simulink model "BimanualHD2LfD_2017a"  (R2017a)
settings: Solver=ode1  StartTime=0.0  StopTime=inf  FixedStep=0.002  RelTol=1e-3  EnableMultiTasking=on
undefined symbols (not defined in the file or in its folder): HIL, qc_get_step_size
libraries: quarc_library x10, simulink_extras x4, dsparch4 x3, simulink x2
(part 2 of 2)

== system BimanualHD2LfD_2017a/HD2 Dynamics/Endonesial I//O/HIL Interfacing/Subsystem1 ==
  Constant2 : Constant  Value=0.01
  Data Type Conversion : DataTypeConversion
  Data Type Conversion1 : DataTypeConversion
  De Bouncer : Subsystem
  De Bouncer1 : Subsystem
  Display : Display
  Display1 : Display
  HIL Read Digital : quarc_library/Data Acquisition/Generic/Immediate I//O/HIL Read Digital  object_name=HIL-1  channels=[0 1 7]  sample_time=qc_get_step_size  active=on  vector_output=off  data_type_mode=Inherit via back propagation  data_type=boolean
      settings: AttributesFormatString=(%<object_name>)
  Left : Outport
  Right : Outport  Port=2
  Touch Sensor : Outport  Port=3
  wires:
  HIL Read Digital/3 -> Touch Sensor/1
  HIL Read Digital/2 -> Display/1, Data Type Conversion1/1
  HIL Read Digital/1 -> Display1/1, Data Type Conversion/1
  Data Type Conversion/1 -> De Bouncer/1(Input)
  Data Type Conversion1/1 -> De Bouncer1/1(Input)
  Constant2/1 -> De Bouncer1/2(debounce_time), De Bouncer/2(debounce_time)
  De Bouncer/1(Output) -> Left/1
  De Bouncer1/1(Output) -> Right/1

== system BimanualHD2LfD_2017a/HD2 Dynamics/Endonesial I//O/HIL Interfacing/Subsystem1/De Bouncer ==
  Input : Inport
  debounce_time : Inport  Port=2
  Data Type Conversion : DataTypeConversion  OutDataTypeStr=int32
  Embedded MATLAB Function : MATLAB Function  TreatAsAtomicUnit=on
  Gain : Gain  Gain=1/qc_get_step_size
  Memory : Memory  InheritSampleTime=on  LinearizeMemory=on  LinearizeAsDelay=on
  Memory1 : Memory  InheritSampleTime=on  LinearizeMemory=on  LinearizeAsDelay=on
  Output : Outport
  wires:
  Embedded MATLAB Function/1(output) -> Memory/1, Output/1
  Embedded MATLAB Function/2(counter) -> Memory1/1
  Memory/1 -> Embedded MATLAB Function/3(prev_output)
  Memory1/1 -> Embedded MATLAB Function/4(prev_counter)
  Input/1 -> Embedded MATLAB Function/1(input)
  debounce_time/1 -> Gain/1
  Data Type Conversion/1 -> Embedded MATLAB Function/2(num_samples)
  Gain/1 -> Data Type Conversion/1

== system BimanualHD2LfD_2017a/HD2 Dynamics/Endonesial I//O/HIL Interfacing/Subsystem1/De Bouncer1 ==
  Input : Inport
  debounce_time : Inport  Port=2
  Data Type Conversion : DataTypeConversion  OutDataTypeStr=int32
  Embedded MATLAB Function : MATLAB Function  TreatAsAtomicUnit=on
  Gain : Gain  Gain=1/qc_get_step_size
  Memory : Memory  InheritSampleTime=on  LinearizeMemory=on  LinearizeAsDelay=on
  Memory1 : Memory  InheritSampleTime=on  LinearizeMemory=on  LinearizeAsDelay=on
  Output : Outport
  wires:
  Gain/1 -> Data Type Conversion/1
  Data Type Conversion/1 -> Embedded MATLAB Function/2(num_samples)
  debounce_time/1 -> Gain/1
  Input/1 -> Embedded MATLAB Function/1(input)
  Memory1/1 -> Embedded MATLAB Function/4(prev_counter)
  Memory/1 -> Embedded MATLAB Function/3(prev_output)
  Embedded MATLAB Function/2(counter) -> Memory1/1
  Embedded MATLAB Function/1(output) -> Output/1, Memory/1

== matlab function BimanualHD2LfD_2017a/GMR/MATLAB Function ==
  data: outputs output; data input; I_vars input; O_vars input; output_var output; model parameter
function [outputs, output_var] = GMR_3DOF (data, I_vars, O_vars, model) 
%#codegen
    [outputs, output_var, ~] = GMR(model, data, I_vars, O_vars);
end

== matlab function BimanualHD2LfD_2017a/Remove Orientation Jump/Remove Orientation Jump ==
  data: signal input; prevSignal input; out output; time input
function out = removeJump(signal, prevSignal, time)
persistent jumpType;
persistent jumpDistance;
persistent jumpCounter;


    if isempty(jumpType) || (time < 0.1)
        jumpType = 0;
        jumpDistance = 0;
        jumpCounter = 0;
    end

    if (signal - prevSignal) < -1
        jumpType = -1;
        jumpCounter = jumpCounter - 1;
        jumpDistance = signal-prevSignal;
        
    elseif (signal - prevSignal) > 1
        jumpType = 1;
        jumpCounter = jumpCounter + 1;
        jumpDistance = signal-prevSignal;
    end
    
    if jumpType == 1
        out = signal - jumpDistance*jumpCounter;
    elseif jumpType == -1
        out = signal + jumpDistance*jumpCounter;
    else
        out = signal;
    end
end

== matlab function BimanualHD2LfD_2017a/Remove Orientation Jump/Remove Orientation Jump1 ==
  data: signal input; prevSignal input; out output; time input
function out = removeJump(signal, prevSignal, time)
persistent jumpType;
persistent jumpDistance;
persistent jumpCounter;


    if isempty(jumpType) || (time < 0.1)
        jumpType = 0;
        jumpDistance = 0;
        jumpCounter = 0;
    end

    if (signal - prevSignal) < -1
        jumpType = -1;
        jumpCounter = jumpCounter - 1;
        jumpDistance = signal-prevSignal;
        
    elseif (signal - prevSignal) > 1
        jumpType = 1;
        jumpCounter = jumpCounter + 1;
        jumpDistance = signal-prevSignal;
    end
    
    if jumpType == 1
        out = signal - jumpDistance*jumpCounter;
    elseif jumpType == -1
        out = signal + jumpDistance*jumpCounter;
    else
        out = signal;
    end
end

== matlab function BimanualHD2LfD_2017a/Kalman Filter ==
  data: x_meas input; DataFilt output
function DataFilt = KalmanFilter(x_meas)
%#codegen
    % Process and sensor noise covariances
    Q =  0.00001;
    R =  1;

    % Initialize estimate and covariance predictions
    persistent x P;
    if (isempty(x) || isempty(P))
        x = -145;
        P = 1;
    end
    P = P + Q;
        
    % Update Kalman gain, and estimate and covariance based on gain
    K = P/(P+R);
    x = x+K*(x_meas-x);
    P = (1-K)*P;
    
    DataFilt = x;
end

== matlab function BimanualHD2LfD_2017a/Remove Orientation Jump/Remove Orientation Jump2 ==
  data: signal input; prevSignal input; out output; time input
function out = removeJump(signal, prevSignal, time)
persistent jumpType;
persistent jumpDistance;
persistent jumpCounter;


    if isempty(jumpType) || (time < 0.1)
        jumpType = 0;
        jumpDistance = 0;
        jumpCounter = 0;
    end

    if (signal - prevSignal) < -1
        jumpType = -1;
        jumpCounter = jumpCounter - 1;
        jumpDistance = signal-prevSignal;
        
    elseif (signal - prevSignal) > 1
        jumpType = 1;
        jumpCounter = jumpCounter + 1;
        jumpDistance = signal-prevSignal;
    end
    
    if jumpType == 1
        out = signal - jumpDistance*jumpCounter;
    elseif jumpType == -1
        out = signal + jumpDistance*jumpCounter;
    else
        out = signal;
    end
end

== matlab function BimanualHD2LfD_2017a/Velpocity Saturation/MATLAB Function ==
  data: v input; v_sat output
function v_sat = saturate(v)
%#codegen
spd = norm(v);
if spd > 99.999
    v_sat = v * 99.999 / spd;
else
    v_sat = v;
end

== matlab function BimanualHD2LfD_2017a/Velocity Decomposition/MATLAB Function ==
  data: velDes input; dirDes output; spdDes output
function [dirDes, spdDes] = fcn(velDes)
%#codegen
    spdDes = norm(velDes);
    if (spdDes > 0)
        dirDes = velDes / spdDes;
    else
        dirDes = [0; 0; 0];
    end
end

== matlab function BimanualHD2LfD_2017a/HD2 Dynamics/Embedded MATLAB Function ==
  data: EmergStop input; out output; u1 input
function out  = fcn(EmergStop,u1)
if EmergStop==0
out=u1;
else
 out=0*u1;
end;

== matlab function BimanualHD2LfD_2017a/HD2 Dynamics/Endonesial I//O/5BAR Linkage Kinematics (Upper)/OMNI Revised Kinematics ==
  data: M input; l1 input; l2 input; p output; l3 input; J output
function [p, J] = Five_Bar_Linkage_Kinematics (M, l1, l2, l3)
	R = l2*cos(M(2)) + l3*cos(M(3));
	x = cos(M(1))*R;
	y = sin(M(1))*R;
	z = l2*sin(M(2)) + l3*sin(M(3)) + l1;
	p = [x y z]';
	J1 = [-sin(M(1))*R      -cos(M(1))*l2*sin(M(2))     -cos(M(1))*l3*sin(M(3))];
	J2 = [cos(M(1))*R       -sin(M(1))*l2*sin(M(2))     -sin(M(1))*l3*sin(M(3))];
	J3 = [0                 l2*cos(M(2))                    l3*cos(M(3))];
	J = [J1;J2;J3];
end

== matlab function BimanualHD2LfD_2017a/HD2 Dynamics/Endonesial I//O/5BAR Linkage Kinematics (Lower)/OMNI Revised Kinematics ==
  data: M input; l1 input; l2 input; p output; l3 input; J output
function [p, J] = Five_Bar_Linkage_Kinematics (M, l1, l2, l3)
% CONSTANTS TO FIX ANGLE OFFSETS, MIGHT NEED TO BE CHANGED (JASON)
e1 = 0.6109; e2 = 1.3963; e3 = 1.6581;

R = l2*cos(M(2)) + l3*cos(M(3));
x = cos(M(1))*R;
y = sin(M(1))*R;
z = l2*sin(M(2)) + l3*sin(M(3)) + l1;
p = [x y z]';
J1 = [-sin(M(1))*R      -cos(M(1))*l2*sin(M(2))     -cos(M(1))*l3*sin(M(3))];
J2 = [cos(M(1))*R       -sin(M(1))*l2*sin(M(2))     -sin(M(1))*l3*sin(M(3))];
J3 = [0                 l2*cos(M(2))                    l3*cos(M(3))];
J = [J1;J2;J3];
end

== matlab function BimanualHD2LfD_2017a/HD2 Dynamics/Endonesial I//O/Calculate Orientation ==
  data: x_upper input; theta_x output; theta_y output; x_lower input; theta_z output; theta_z_p input; counterNew output; counterOld input; theta_z_out output
function [theta_x, theta_y, theta_z, counterNew, theta_z_out] = ...
	fcn(x_upper, x_lower, theta_z_p, counterOld)
	% This block supports the Embedded MATLAB subset.
	% See the help menu for details. 

	theta_x = atan2(x_upper(3) - x_lower(3), x_upper(2) - x_lower(2));
	theta_y = atan2(x_upper(1) - x_lower(1), x_upper(3) - x_lower(3));
	theta_z = atan2(x_upper(2) - x_lower(2), x_upper(1) - x_lower(1));

	counterNew = counterOld;

	if theta_z >= 0
		F1 = mod(theta_z, 2*pi);
		theta_z = F1;
	else
		F1 = mod(theta_z, -2*pi) + 2*pi;
		theta_z = F1;
	end

	d_theta_z = theta_z_p - theta_z;

	if abs(d_theta_z) > 5
		if d_theta_z > 0
		counterNew = counterOld + 1;
		end
		if d_theta_z < 0
		counterNew = counterOld - 1;
		end
	end
 
	theta_z_out = theta_z + 2*pi*counterNew;
end

== matlab function BimanualHD2LfD_2017a/HD2 Dynamics/Endonesial I//O/HD^2 New Kin new frame/New Numerical Kin ==
  data: q input; pos output; or output; ang output; poses output; Trans output; nn output; x output
 function [pos, or ,ang , poses, Trans, nn, x] = HDsquared_forwardkin(q)

    x = [0 0 0 0]';
    l = [220 40 125 22.25 250];
    ang = [0 0 0];
    
  
    nn = 0;
    while ( (norm(fnum(q,x,l)) > 0.0001) && nn <20)
      nn = nn+1;
        x = x - inv(Jnum(q,x,l))*fnum(q,x,l)';
    end
    
    
    
    pos = handlePos(q,x,l)';
    or = handleOr(q,x,l);
     
%     yaw = atan2 (or(2,1),or(1,1));   %AA
%     roll = atan2 ( or(3,2),or(3,3) );  %AA
%     pitch = atan2( -or(3,1), sqrt(  or(3,2)^2 + or(3,3)^2 ) ); %AA
%     
%     ang = [yaw;pitch;roll];  %AA
    
    pos_top = 250/2*(or(:,3))+pos;
    pos_bottom = -250/2*(or(:,3))+pos;
    poses = [pos_top;pos_bottom];
    
    Trans1 = cat(2,or,pos);
    Trans = cat(1,Trans1,[0 0 0 1]);
    
end


function val = fnum(q,x,l)

val = zeros(1,4); %AA
    q1 = q(1);
    q2 = q(2);
    q3 = q(3);
    q4 = q(4);
    q5 = q(5);
    q6 = q(6);
    
    l1 = l(1);
    l2 = l(2);
    l3 = l(3);
    l4 = l(4);
    l5 = l(5);
    
    alpha_u = x(1);
    theta_u = x(2);
    alpha_l = x(3);
    theta_l = x(4);
    
    t1 = pi / 0.4e1;
    t3 = cos(t1 + q1);
    t4 = sin(alpha_u);
    t5 = t3 * t4;
    t7 = cos(-t1 + q1);
    t8 = sin(theta_u);
    t9 = t7 * t8;
    t10 = cos(alpha_u);
    t11 = t9 * t10;
    t13 = cos(t1 + q4);
    t14 = sin(alpha_l);
    t15 = t13 * t14;
    t17 = cos(-t1 + q4);
    t18 = sin(theta_l);
    t19 = t17 * t18;
    t20 = cos(alpha_l);
    t21 = t19 * t20;
    t23 = cos(q3);
    t24 = t23 * t7;
    t25 = t24 * t4;
    t28 = sin(q3);
    t29 = cos(theta_u);
    t31 = t23 * t3 * t8 + t28 * t29;
    t32 = t31 * t10;
    t33 = cos(q6);
    t34 = t33 * t17;
    t35 = t34 * t14;
    t38 = sin(q6);
    t39 = cos(theta_l);
    t41 = t33 * t13 * t18 + t38 * t39;
    t42 = t41 * t20;
    t45 = cos(-t1 + q2);
    t56 = cos(-t1 + q5);
    t68 = cos(t1 + q2);
    t80 = cos(t1 + q5);
    val(1) = t5 + t11 - t15 - t21;
    val(2) = -t25 + t32 + t35 - t42;
    val(3) = t45 * l1 - t3 * l1 + (-t3 * t10 + t9 * t4) * l4 - (t5 + t11) * l5 / 0.2e1 - t56 * l1 + t13 * l1 - (-t13 * t20 + t19 * t14) * l4 - (t15 + t21) * l5 / 0.2e1;
    val(4) = t23 * t68 * l1 + t24 * l1 + (t24 * t10 + t31 * t4) * l4 - (-t25 + t32) * l5 / 0.2e1 - t33 * t80 * l1 - t34 * l1 - (t34 * t20 + t41 * t14) * l4 - (-t35 + t42) * l5 / 0.2e1;

end



function val2 = Jnum(q,x,l)
val2 = zeros(4,4); %AA
    q1 = q(1);
    q2 = q(2);
    q3 = q(3);
    q4 = q(4);
    q5 = q(5);
    q6 = q(6);
    
    l1 = l(1);
    l2 = l(2);
    l3 = l(3);
    l4 = l(4);
    l5 = l(5);
    
    
    alpha_u = x(1);
    theta_u = x(2);
    alpha_l = x(3);
    theta_l = x(4);
    
    t1 = pi / 0.4e1;
    t3 = cos(t1 + q1);
    t4 = cos(alpha_u);
    t7 = cos(-t1 + q1);
    t8 = sin(theta_u);
    t9 = t7 * t8;
    t10 = sin(alpha_u);
    t12 = t3 * t4 - t9 * t10;
    t13 = cos(theta_u);
    t14 = t7 * t13;
    t17 = cos(t1 + q4);
    t18 = cos(alpha_l);
    t21 = cos(-t1 + q4);
    t22 = sin(theta_l);
    t23 = t21 * t22;
    t24 = sin(alpha_l);
    t26 = -t17 * t18 + t23 * t24;
    t27 = cos(theta_l);
    t28 = t21 * t27;
    t30 = cos(q3);
    t31 = t30 * t7;
    t33 = t30 * t3;
    t35 = sin(q3);
    t37 = t33 * t8 + t35 * t13;
    t39 = -t31 * t4 - t37 * t10;
    t42 = t33 * t13 - t35 * t8;
    t43 = t42 * t4;
    t44 = cos(q6);
    t45 = t44 * t21;
    t47 = t44 * t17;
    t49 = sin(q6);
    t51 = t47 * t22 + t49 * t27;
    t53 = t45 * t18 + t51 * t24;
    t56 = t47 * t27 - t49 * t22;
    t57 = t56 * t18;
    val2(1,1) = t12;
    val2(1,2) = t14 * t4;
    val2(1,3) = t26;
    val2(1,4) = -t28 * t18;
    val2(2,1) = t39;
    val2(2,2) = t43;
    val2(2,3) = t53;
    val2(2,4) = -t57;
    val2(3,1) = (t3 * t10 + t9 * t4) * l4 - t12 * l5 / 0.2e1;
    val2(3,2) = t14 * t10 * l4 - t14 * t4 * l5 / 0.2e1;
    val2(3,3) = -(t17 * t24 + t23 * t18) * l4 + t26 * l5 / 0.2e1;
    val2(3,4) = -t28 * t24 * l4 - t28 * t18 * l5 / 0.2e1;
    val2(4,1) = (-t31 * t10 + t37 * t4) * l4 - t39 * l5 / 0.2e1;
    val2(4,2) = t42 * t10 * l4 - t43 * l5 / 0.2e1;
    val2(4,3) = -(-t45 * t24 + t51 * t18) * l4 + t53 * l5 / 0.2e1;
    val2(4,4) = -t56 * t24 * l4 - t57 * l5 / 0.2e1;

end

function val3 = handlePos(q,x,l)
 val3 = zeros(1,3);   %AA
    q1 = q(1);
    q2 = q(2);
    q3 = q(3);
    q4 = q(4);
    q5 = q(5);
    q6 = q(6);
    
    l1 = l(1);
    l2 = l(2);
    l3 = l(3);
    l4 = l(4);
    l5 = l(5);
    
    
    alpha_u = x(1);
    theta_u = x(2);
    alpha_l = x(3);
    theta_l = x(4);

    t1 = pi / 0.4e1;
    t3 = cos(-t1 + q2);
    t6 = cos(t1 + q1);
    t8 = cos(alpha_u);
    t11 = cos(-t1 + q1);
    t12 = sin(theta_u);
    t13 = t11 * t12;
    t14 = sin(alpha_u);
    t24 = cos(q3);
    t26 = cos(t1 + q2);
    t29 = t24 * t11;
    t34 = sin(q3);
    t35 = cos(theta_u);
    t37 = t24 * t6 * t12 + t34 * t35;
    t49 = t34 * t11;
    t55 = -t34 * t6 * t12 + t24 * t35;
    val3(1) = t3 * l1 - t6 * l1 + (-t6 * t8 + t13 * t14) * l4 - (t6 * t14 + t13 * t8) * l5 / 0.2e1;
    val3(2) = t24 * t26 * l1 + t29 * l1 + (t29 * t8 + t37 * t14) * l4 - (-t29 * t14 + t37 * t8) * l5 / 0.2e1;
    val3(3) = l3 - t34 * t26 * l1 - t49 * l1 + (-t49 * t8 + t55 * t14) * l4 - (t49 * t14 + t55 * t8) * l5 / 0.2e1;

end

function val4 = handleOr(q,x,l)
  val4 = zeros(3,3);  %AA 
    q1 = q(1);
    q2 = q(2);
    q3 = q(3);
    q4 = q(4);
    q5 = q(5);
    q6 = q(6);
    q7 = q(7);
    
    l1 = l(1);
    l2 = l(2);
    l3 = l(3);
    l4 = l(4);
    l5 = l(5);
    
    
    alpha_u = x(1);
    theta_u = x(2);
    alpha_l = x(3);
    theta_l = x(4);
    
    t1 = pi / 0.4e1;
    t3 = cos(-t1 + q1);
    t4 = cos(theta_u);
    t5 = t3 * t4;
    t6 = cos(q7);
    t9 = cos(t1 + q1);
    t10 = cos(alpha_u);
    t12 = sin(theta_u);
    t13 = t3 * t12;
    t14 = sin(alpha_u);
    t16 = -t9 * t10 + t13 * t14;
    t17 = sin(q7);
    t26 = cos(q3);
    t27 = t26 * t9;
    t29 = sin(q3);
    t31 = t27 * t4 - t29 * t12;
    t33 = t26 * t3;
    t37 = t27 * t12 + t29 * t4;
    t39 = t33 * t10 + t37 * t14;
    t48 = t29 * t9;
    t51 = -t48 * t4 - t26 * t12;
    t53 = t29 * t3;
    t57 = -t48 * t12 + t26 * t4;
    t59 = -t53 * t10 + t57 * t14;
    val4(1,1) = t5 * t6 + t16 * t17;
    val4(1,2) = -t5 * t17 + t16 * t6;
    val4(1,3) = t9 * t14 + t13 * t10;
    val4(2,1) = t31 * t6 + t39 * t17;
    val4(2,2) = -t31 * t17 + t39 * t6;
    val4(2,3) = -t33 * t14 + t37 * t10;
    val4(3,1) = t51 * t6 + t59 * t17;
    val4(3,2) = -t51 * t17 + t59 * t6;
    val4(3,3) = t53 * t14 + t57 * t10;

end

== matlab function BimanualHD2LfD_2017a/HD2 Dynamics/Endonesial I//O/HIL Interfacing/Subsystem1/De Bouncer/Embedded MATLAB Function ==
  data: input input; num_samples input int32; output output; prev_output input; prev_counter input int32; counter output int32
function [output, counter] = de_bouncer(input,  num_samples,prev_output, prev_counter)
if (prev_output ~= input)
    % Change detected
    counter = prev_counter - 1;
    if (counter == 0)
        output = input;
    else
        output = prev_output;
    end
else
    counter = num_samples;
    output = prev_output;
end

== matlab function BimanualHD2LfD_2017a/HD2 Dynamics/Endonesial I//O/HIL Interfacing/Subsystem1/De Bouncer1/Embedded MATLAB Function ==
  data: input input; num_samples input int32; output output; prev_output input; prev_counter input int32; counter output int32
function [output, counter] = de_bouncer(input,  num_samples,prev_output, prev_counter)
if (prev_output ~= input)
    % Change detected
    counter = prev_counter - 1;
    if (counter == 0)
        output = input;
    else
        output = prev_output;
    end
else
    counter = num_samples;
    output = prev_output;
end

== matlab function BimanualHD2LfD_2017a/HD2 Dynamics/Endonesial I//O/Torque to Force ==
  data: x_lower input; F_upper output; F_lower output; x_upper input; tau input; l11 input; l22 input
function [F_upper,F_lower] = fcn(x_lower,x_upper,tau,l11,l22)
% This block supports the Embedded MATLAB subset.
% See the help menu for details. 


%Initialization
F_upper=zeros(3,1);
F_lower=zeros(3,1);

if l11 == 0 
    sg1 = 1;
else
    sg1= sign(l11);
end

if l22 == 0 
    sg2 = 1;
else
    sg2= sign(l22);
end



if abs(l11)<0.005 
    l1 = 0.005 * sg1;
else
    l1= l11;
end

if abs(l22)<0.005 
    l2 = 0.005 * sg2;
else
    l2= l22;
end
%%%%%%%%%%%%%%%%%%%%%%%%%%%%

link = sqrt (  (x_upper(3)-x_lower(3))^2 + (x_upper(1)-x_lower(1))^2  + (x_upper(2)-x_lower(2))^2  );
unitvec = (x_upper - x_lower)/link;
F_upper = ( cross (tau,unitvec))/2/l1;
F_lower = - ( cross (tau,unitvec))/2/l2;


% link = sqrt (  (x_upper(3)-x_lower(3))^2 + (x_upper(1)-x_lower(1))^2  + (x_upper(2)-x_lower(2))^2  );
% unitvec = (x_upper - x_lower)/link;
% F_upper = 2/link * ( cross (tau,unitvec));
% F_lower = - F_upper;
% 

% link = sqrt (  (x_upper(3)-x_lower(3))^2 + (x_upper(1)-x_lower(1))^2  + (x_upper(2)-x_lower(2))^2  );
% unitvec = (x_lower - x_upper)/link;
% F_upper = (5/link * ( cross (tau,unitvec)));
% F_lower = F_upper/6;

== matlab function BimanualHD2LfD_2017a/HD2 Dynamics/Endonesial I//O/Calculate Mean Position ==
  data: x_mean output; x input; l1 input
function x_mean  = mean1(x,l1)
% This block supports the Embedded MATLAB subset.
% See the help menu for details. 
% link = .175;%25;
% l2=link - l1;
% 
% x_mean=zeros(3,1);
% x_mean(1)=(l2*x(1)+l1*x(4))/link;
% x_mean(2)=(l2*x(2)+l1*x(5))/link;
% x_mean(3)=(l2*x(3)+l1*x(6))/link;

x_mean=zeros(3,1);
x_mean(1)=(x(1)+x(4))/2;
x_mean(2)=(x(2)+x(5))/2;
x_mean(3)=(x(3)+x(6))/2;
